simulink model "obs_com_filtro_2020"  (R2020b)
settings: Solver=VariableStepAuto  StartTime=0.0  StopTime=600  RelTol=1e-3
model workspace (MAT data in the model file):
  Td = 2
  std_dev = 0.08
values from neighbouring files (symbols this model uses):
  K = 0.002677    [run_and_calculate.m]
  T = 0.5    [run_and_calculate.m]
libraries: cstblocks x20
settings Model: Creator=Gabriel Vieira  LastModifiedBy=Gabriel Vieira
settings DebuggingCC: SFMachineParentedDataDiag=error

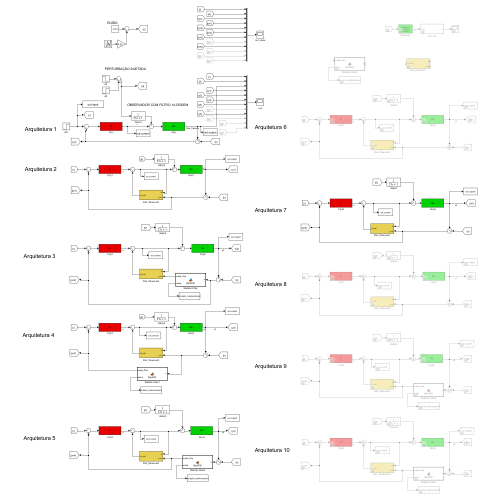
[thumbnail: Simulink's stored preview of the top-level diagram]
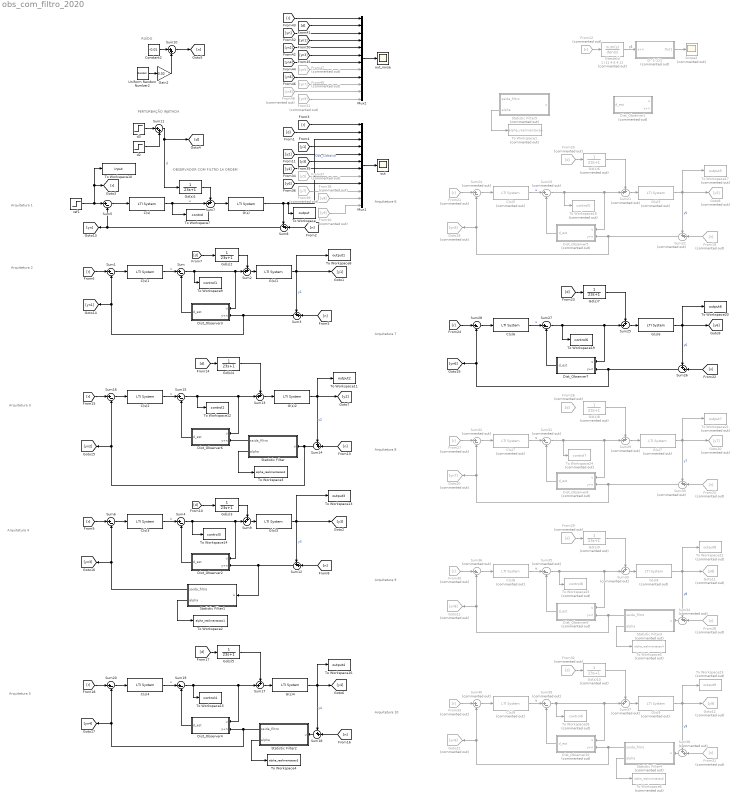
== system obs_com_filtro_2020 ==
  note: RUÍDO
  note: OBSERVADOR COM FILTRO 1A ORDEM
  note: PERTURBAÇÃO INJETADA
  note: Arquitetura 1
  note: Arquitetura 2
  note: Arquitetura 3
  note: Arquitetura 4
  note: Arquitetura 5
  note: Arquitetura 6
  note: Arquitetura 7
  note: Arquitetura 8
  note: Arquitetura 9
  note: Arquitetura 10
  C(s){,1..4,6} (6 alike) : cstblocks/LTI System  sys=C  IC=[]
  C(s){5,7..9} (4 alike) : cstblocks/LTI System  Commented=on  sys=C  IC=[]
  Constant2 : Constant  Value=-0.01
  Dist_Observer1 : Subsystem  Commented=on  mask{std_dev=std_dev}
      mask prompts: std_dev "Noise Std Deviation (std_dev)"
  Dist_Observer10 : Subsystem  Commented=on  mask{Td=Td, std_dev=std_dev}
      mask prompts: Td "Filter time cte (Td)"; std_dev "Noised Std Derivation"
  Dist_Observer2 : Subsystem  mask{Td=Td}
      mask prompts: Td "Filter time cte (Td)"
  Dist_Observer3 : Subsystem  mask{Td=Td}
      mask prompts: Td "Filter time cte (Td)"
  Dist_Observer4 : Subsystem  mask{Td=Td}
      mask prompts: Td "Filter time cte (Td)"
  Dist_Observer5 : Subsystem  Commented=on  mask{Td=Td, std_dev=std_dev}
      mask prompts: Td "Filter time cte (Td)"; std_dev "Noised Std Derivation"
  Dist_Observer6 : Subsystem  mask{Td=Td}
      mask prompts: Td "Filter time cte (Td)"
  Dist_Observer7 : Subsystem  mask{Td=Td, std_dev=std_dev}
      mask prompts: Td "Filter time cte (Td)"; std_dev "Noised Std Derivation"
  Dist_Observer8 : Subsystem  Commented=on  mask{std_dev=std_dev}
      mask prompts: std_dev "Noised Std Derivation"
  Dist_Observer9 : Subsystem  Commented=on  mask{Td=Td, std_dev=std_dev}
      mask prompts: Td "Filter time cte (Td)"; std_dev "Noised Std Derivation"
  From{12,21,27,30,33} (5 alike) : From  Commented=on  GotoTag=r
  From{19,25,28,31} (4 alike) : From  Commented=on  GotoTag=n
  From{20,26,29,32} (4 alike) : From  Commented=on  GotoTag=d
  From37 : From  Commented=on  GotoTag=y5
  From38 : From  Commented=on  GotoTag=y8
  From39 : From  Commented=on  GotoTag=y7
  From40 : From  Commented=on  GotoTag=y9
  From47 : From  Commented=on  GotoTag=yn5
  From48 : From  Commented=on  GotoTag=yn8
  From49 : From  Commented=on  GotoTag=yn7
  From51 : From  Commented=on  GotoTag=yn9
  G(s){,1..4,6} (6 alike) : cstblocks/LTI System  sys=Gs  IC=[]
  G(s){5,7..9} (4 alike) : cstblocks/LTI System  Commented=on  sys=Gs  IC=[]
  "G^{-1}1" : Subsystem  Commented=on
  Gain2 : Gain  Gain=0.02
  Gd(s){1..5,7} (6 alike) : TransferFcn  Numerator=1  Denominator=[23 1]
  Gd(s){6,8..10} (4 alike) : TransferFcn  Commented=on  Numerator=1  Denominator=[23 1]
  Goto10 : Goto  Commented=on  GotoTag=y7
  Goto11 : Goto  Commented=on  GotoTag=y8
  Goto12 : Goto  Commented=on  GotoTag=y9
  Goto18 : Goto  Commented=on  GotoTag=yn5
  Goto20 : Goto  Commented=on  GotoTag=yn7
  Goto21 : Goto  Commented=on  GotoTag=yn8
  Goto22 : Goto  Commented=on  GotoTag=yn9
  Goto8 : Goto  Commented=on  GotoTag=y5
  Gteste(s) : TransferFcn  Commented=on  Numerator=1  Denominator=[1 4 6 4 1]
  Mux1 : Mux  Inputs=12
  Mux2 : Mux  Inputs=12
  Scope2 : Scope  Commented=on
  Statistic Filter : MATLAB Function  TreatAsAtomicUnit=on  mask{std_dev=0.5}
      mask prompts: std_dev "Noise Std Deviation (std_dev)"
  Statistic Filter1 : MATLAB Function  TreatAsAtomicUnit=on  mask{std_dev=0.5}
      mask prompts: std_dev "Noise Std Deviation (std_dev)"
  Statistic Filter2 : MATLAB Function  TreatAsAtomicUnit=on  mask{std_dev=0.5}
      mask prompts: std_dev "Noise Std Deviation (std_dev)"
  Statistic Filter3 : MATLAB Function  Commented=on  TreatAsAtomicUnit=on  mask{std_dev=0.5}
      mask prompts: std_dev "Noise Std Deviation (std_dev)"
  Statistic Filter4 : MATLAB Function  Commented=on  TreatAsAtomicUnit=on  mask{std_dev=0.5}
      mask prompts: std_dev "Noise Std Deviation (std_dev)"
  Statistic Filter5 : MATLAB Function  Commented=on  TreatAsAtomicUnit=on  mask{std_dev=0.5}
      mask prompts: std_dev "Noise Std Deviation (std_dev)"
  Sum{,1,4..6,15..16,19..20,27..28} (11 alike) : Sum  Inputs=|+-
  Sum10 : Sum  Inputs=|++
  Sum11 : Sum  Inputs=|++
  Sum{2..3,7..9,12..14,17..18,25..26} (12 alike) : Sum  Inputs=++|
  Sum{21..22,29..30,33..34,37..38} (8 alike) : Sum  Commented=on  Inputs=++|
  Sum{23..24,31..32,35..36,39..40} (8 alike) : Sum  Commented=on  Inputs=|+-
  To Workspace : ToWorkspace  VariableName=output  SaveFormat=Timeseries  SampleTime=-1
  To Workspace1 : ToWorkspace  Commented=on  VariableName=alpha_realimentacao  SaveFormat=Timeseries  SampleTime=-1
  To Workspace10 : ToWorkspace  VariableName=input  SaveFormat=Timeseries  SampleTime=-1
  To Workspace11 : ToWorkspace  VariableName=output2  SaveFormat=Timeseries  SampleTime=-1
  To Workspace12 : ToWorkspace  VariableName=control2  SaveFormat=Timeseries  SampleTime=-1
  To Workspace13 : ToWorkspace  VariableName=output3  SaveFormat=Timeseries  SampleTime=-1
  To Workspace14 : ToWorkspace  VariableName=control3  SaveFormat=Timeseries  SampleTime=-1
  To Workspace15 : ToWorkspace  VariableName=control4  SaveFormat=Timeseries  SampleTime=-1
  To Workspace16 : ToWorkspace  VariableName=output4  SaveFormat=Timeseries  SampleTime=-1
  To Workspace17 : ToWorkspace  Commented=on  VariableName=output5  SaveFormat=Timeseries  SampleTime=-1
  To Workspace18 : ToWorkspace  Commented=on  VariableName=control5  SaveFormat=Timeseries  SampleTime=-1
  To Workspace19 : ToWorkspace  VariableName=control6  SaveFormat=Timeseries  SampleTime=-1
  To Workspace2 : ToWorkspace  VariableName=alpha_realimentacao1  SaveFormat=Timeseries  SampleTime=-1
  To Workspace20 : ToWorkspace  VariableName=output6  SaveFormat=Timeseries  SampleTime=-1
  To Workspace21 : ToWorkspace  Commented=on  VariableName=output7  SaveFormat=Timeseries  SampleTime=-1
  To Workspace22 : ToWorkspace  Commented=on  VariableName=output8  SaveFormat=Timeseries  SampleTime=-1
  To Workspace23 : ToWorkspace  Commented=on  VariableName=output9  SaveFormat=Timeseries  SampleTime=-1
  To Workspace24 : ToWorkspace  Commented=on  VariableName=control7  SaveFormat=Timeseries  SampleTime=-1
  To Workspace25 : ToWorkspace  Commented=on  VariableName=control8  SaveFormat=Timeseries  SampleTime=-1
  To Workspace26 : ToWorkspace  Commented=on  VariableName=control9  SaveFormat=Timeseries  SampleTime=-1
  To Workspace3 : ToWorkspace  VariableName=alpha_realimentacao2  SaveFormat=Timeseries  SampleTime=-1
  To Workspace4 : ToWorkspace  VariableName=alpha_realimentacao3  SaveFormat=Timeseries  SampleTime=-1
  To Workspace5 : ToWorkspace  Commented=on  VariableName=alpha_realimentacao4  SaveFormat=Timeseries  SampleTime=-1
  To Workspace6 : ToWorkspace  Commented=on  VariableName=alpha_realimentacao6  SaveFormat=Timeseries  SampleTime=-1
  To Workspace7 : ToWorkspace  VariableName=control  SaveFormat=Timeseries  SampleTime=-1
  To Workspace8 : ToWorkspace  VariableName=output1  SaveFormat=Timeseries  SampleTime=-1
  To Workspace9 : ToWorkspace  VariableName=control1  SaveFormat=Timeseries  SampleTime=-1
  Uniform Random Number2 : UniformRandomNumber  SampleTime=0.01
  d2 : Step  Time=150  SampleTime=0
  d3 : Step  Time=200  After=-1  SampleTime=0
  out : Scope
  out_noise : Scope
  ref1 : Step  Time=50  SampleTime=0
  wires:
  Sum10/1 -> [n]
  Constant2/1 -> Sum10/1
  Sum5/1 -> C(s)/1
  d2/1 -> Sum11/2
  C(s)/1 -> To Workspace7/1, Sum7/2  "u"
  Gain2/1 -> Sum10/2
  ref1/1 -> To Workspace10/1, [r], Sum5/1
  Uniform Random Number2/1 -> Gain2/1
  Mux1/1 -> out/1
  Sum7/1 -> G(s)/1
  Sum11/1 -> [d], Gd(s)1/1  "d"
  [r] -> Mux1/1
  Gd(s)1/1 -> Sum7/1
  [n] -> Sum8/2
  d3/1 -> Sum11/1
  G(s)/1 -> Sum8/1, To Workspace/1, Mux1/3  "Obs_Classico"
  Sum8/1 -> [yn], Sum5/2
  [d] -> Mux1/2
  [n] -> Sum3/2
  Gd(s)2/1 -> Sum2/1
  Sum2/1 -> G(s)1/1
  Sum1/1 -> C(s)1/1
  [r] -> Sum1/1
  [d] -> Gd(s)2/1
  C(s)1/1 -> Sum/1  "u"
  Sum/1 -> To Workspace9/1, Dist_Observer3/1(u), Sum2/2
  Sum3/1 -> Dist_Observer3/2(y+n), [yn1], Sum1/2
  Dist_Observer3/1(d_est) -> Sum/2
  G(s)1/1 -> To Workspace8/1, [y1], Sum3/1  "y1"
  [y1] -> Mux1/4
  Statistic Filter5/2(alpha) -> To Workspace1/1
  Sum9/1 -> G(s)3/1
  Gd(s)3/1 -> Sum9/1
  G(s)3/1 -> To Workspace13/1, [y3], Sum12/1  "y3"
  Sum4/1 -> To Workspace14/1, Dist_Observer2/1(u), Sum9/2
  [r] -> Sum6/1
  [d] -> Gd(s)3/1
  C(s)3/1 -> Sum4/1  "u"
  Dist_Observer2/1(d_est) -> Sum4/2
  Sum6/1 -> C(s)3/1
  [n] -> Sum12/2
  Sum12/1 -> Statistic Filter1/1(u), Dist_Observer2/2(y+n)
  Statistic Filter1/2(alpha) -> To Workspace2/1
  [y2] -> Mux1/5
  Gteste(s)/1 -> "G^{-1}1"/1(y+n)  "y1"
  From12/1 -> Gteste(s)/1
  "G^{-1}1"/1(Out1) -> Scope2/1
  Sum15/1 -> To Workspace12/1, Dist_Observer6/1(u), Sum13/2
  [d] -> Gd(s)4/1
  Sum13/1 -> G(s)2/1
  Gd(s)4/1 -> Sum13/1
  [n] -> Sum14/2
  G(s)2/1 -> Sum14/1, To Workspace11/1, [y2]  "y2"
  Statistic Filter/2(alpha) -> To Workspace3/1
  Sum16/1 -> C(s)2/1
  Dist_Observer6/1(d_est) -> Sum15/2
  C(s)2/1 -> Sum15/1  "u"
  Statistic Filter/1(saida_filtro) -> Dist_Observer6/2(y+n)
  [r] -> Sum16/1
  Dist_Observer4/1(d_est) -> Sum19/2
  [r] -> Sum20/1
  Sum17/1 -> G(s)4/1
  Sum18/1 -> Statistic Filter2/1(u)
  Statistic Filter2/2(alpha) -> To Workspace4/1
  G(s)4/1 -> To Workspace16/1, [y4], Sum18/1  "y4"
  [d] -> Gd(s)5/1
  Sum20/1 -> C(s)4/1
  C(s)4/1 -> Sum19/1  "u"
  Sum19/1 -> To Workspace15/1, Dist_Observer4/1(u), Sum17/2
  Gd(s)5/1 -> Sum17/1
  [n] -> Sum18/2
  Sum23/1 -> To Workspace18/1, Dist_Observer5/1(u), Sum21/2
  From19/1 -> Sum22/2
  Gd(s)6/1 -> Sum21/1
  Sum24/1 -> C(s)5/1
  From20/1 -> Gd(s)6/1
  C(s)5/1 -> Sum23/1  "u"
  G(s)5/1 -> To Workspace17/1, Goto8/1, Sum22/1  "y5"
  Dist_Observer5/1(d_est) -> Sum23/2
  Sum21/1 -> G(s)5/1
  From21/1 -> Sum24/1
  Gd(s)7/1 -> Sum25/1
  Sum27/1 -> To Workspace19/1, Dist_Observer7/1(u), Sum25/2
  [n] -> Sum26/2
  G(s)6/1 -> To Workspace20/1, [y6], Sum26/1  "y6"
  Sum28/1 -> C(s)6/1
  C(s)6/1 -> Sum27/1  "u"
  [r] -> Sum28/1
  Dist_Observer7/1(d_est) -> Sum27/2
  [d] -> Gd(s)7/1
  Sum25/1 -> G(s)6/1
  Sum31/1 -> Dist_Observer8/1(u), Sum29/2, To Workspace24/1
  Gd(s)8/1 -> Sum29/1
  Dist_Observer8/1(d_est) -> Sum31/2
  From27/1 -> Sum32/1
  C(s)7/1 -> Sum31/1  "u"
  Sum32/1 -> C(s)7/1
  From25/1 -> Sum30/2
  G(s)7/1 -> To Workspace21/1, Goto10/1, Sum30/1  "y7"
  Sum29/1 -> G(s)7/1
  Sum38/1 -> Statistic Filter4/1(u)
  Statistic Filter4/2(alpha) -> To Workspace6/1
  Sum39/1 -> To Workspace26/1, Dist_Observer10/1(u), Sum37/2
  Gd(s)10/1 -> Sum37/1
  Dist_Observer10/1(d_est) -> Sum39/2
  G(s)9/1 -> To Workspace23/1, Goto12/1, Sum38/1  "y9"
  From31/1 -> Sum38/2
  Sum34/1 -> Statistic Filter3/1(u)
  Sum40/1 -> C(s)9/1
  C(s)9/1 -> Sum39/1  "u"
  Statistic Filter3/2(alpha) -> To Workspace5/1
  Gd(s)9/1 -> Sum33/1
  Sum35/1 -> To Workspace25/1, Dist_Observer9/1(u), Sum33/2
  From28/1 -> Sum34/2
  G(s)8/1 -> To Workspace22/1, Goto11/1, Sum34/1  "y8"
  From30/1 -> Sum36/1
  From33/1 -> Sum40/1
  Dist_Observer9/1(d_est) -> Sum35/2
  From29/1 -> Gd(s)9/1
  Sum33/1 -> G(s)8/1
  Sum37/1 -> G(s)9/1
  Sum36/1 -> C(s)8/1
  C(s)8/1 -> Sum35/1  "u"
  From32/1 -> Gd(s)10/1
  [y3] -> Mux1/6
  [y4] -> Mux1/7
  From37/1 -> Mux1/8
  [y6] -> Mux1/9
  From39/1 -> Mux1/10
  From38/1 -> Mux1/11
  From40/1 -> Mux1/12
  From51/1 -> Mux2/12
  From48/1 -> Mux2/11
  [yn6] -> Mux2/9
  From49/1 -> Mux2/10
  [yn3] -> Mux2/6
  [yn1] -> Mux2/4
  From47/1 -> Mux2/8
  [r] -> Mux2/1
  [yn4] -> Mux2/7
  [d] -> Mux2/2
  Mux2/1 -> out_noise/1
  [yn2] -> Mux2/5
  [yn] -> Mux2/3
  Sum14/1 -> Statistic Filter/1(u), [yn2], Sum16/2
  Statistic Filter1/1(saida_filtro) -> [yn3], Sum6/2
  Statistic Filter2/1(saida_filtro) -> Dist_Observer4/2(y+n), [yn4], Sum20/2
  Sum22/1 -> Dist_Observer5/2(y+n), Goto18/1, Sum24/2
  Sum26/1 -> Dist_Observer7/2(y+n), [yn6], Sum28/2
  Sum30/1 -> Dist_Observer8/2(y+n), Goto20/1, Sum32/2
  Statistic Filter3/1(saida_filtro) -> Dist_Observer9/2(y+n), Goto21/1, Sum36/2
  Statistic Filter4/1(saida_filtro) -> Dist_Observer10/2(y+n), Goto22/1, Sum40/2

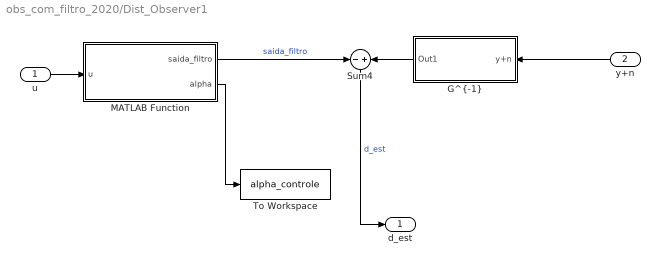
== system obs_com_filtro_2020/Dist_Observer1 ==
  u : Inport
  y+n : Inport  Port=2
  "G^{-1}" : Subsystem
  MATLAB Function : MATLAB Function  TreatAsAtomicUnit=on
  Sum4 : Sum  Inputs=-|+
  To Workspace : ToWorkspace  VariableName=alpha_controle  SaveFormat=Timeseries  SampleTime=-1
  d_est : Outport
  wires:
  MATLAB Function/1(saida_filtro) -> Sum4/1  "saida_filtro"
  Sum4/1 -> d_est/1  "d_est"
  u/1 -> MATLAB Function/1(u)
  "G^{-1}"/1(Out1) -> Sum4/2
  MATLAB Function/2(alpha) -> To Workspace/1
  y+n/1 -> "G^{-1}"/1(y+n)

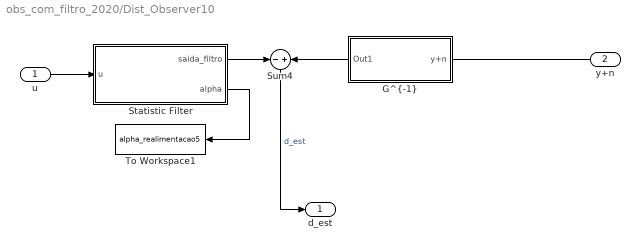
== system obs_com_filtro_2020/Dist_Observer10 ==
  u : Inport
  y+n : Inport  Port=2
  "G^{-1}" : Subsystem
  Statistic Filter : MATLAB Function  TreatAsAtomicUnit=on  mask{std_dev=0.5}
      mask prompts: std_dev "Noise Std Deviation (std_dev)"
  Sum4 : Sum  Inputs=-|+
  To Workspace1 : ToWorkspace  VariableName=alpha_realimentacao5  SaveFormat=Timeseries  SampleTime=-1
  d_est : Outport
  wires:
  Statistic Filter/1(saida_filtro) -> Sum4/1
  Sum4/1 -> d_est/1  "d_est"
  u/1 -> Statistic Filter/1(u)
  "G^{-1}"/1(Out1) -> Sum4/2
  y+n/1 -> ?
  Statistic Filter/2(alpha) -> To Workspace1/1

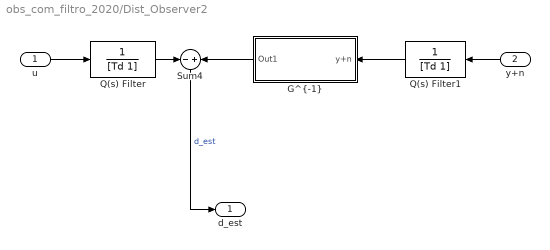
== system obs_com_filtro_2020/Dist_Observer2 ==
  u : Inport
  y+n : Inport  Port=2
  "G^{-1}" : Subsystem
  Q(s) Filter : TransferFcn  Denominator=[Td 1]
  Q(s) Filter1 : TransferFcn  Denominator=[Td 1]
  Sum4 : Sum  Inputs=-|+
  d_est : Outport
  wires:
  Q(s) Filter/1 -> Sum4/1
  Sum4/1 -> d_est/1  "d_est"
  u/1 -> Q(s) Filter/1
  "G^{-1}"/1(Out1) -> Sum4/2
  Q(s) Filter1/1 -> "G^{-1}"/1(y+n)
  y+n/1 -> Q(s) Filter1/1

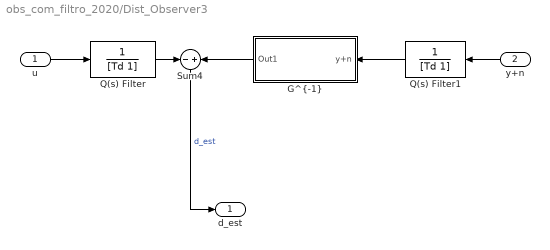
== system obs_com_filtro_2020/Dist_Observer3 ==
  u : Inport
  y+n : Inport  Port=2
  "G^{-1}" : Subsystem
  Q(s) Filter : TransferFcn  Denominator=[Td 1]
  Q(s) Filter1 : TransferFcn  Denominator=[Td 1]
  Sum4 : Sum  Inputs=-|+
  d_est : Outport
  wires:
  Q(s) Filter/1 -> Sum4/1
  Sum4/1 -> d_est/1  "d_est"
  u/1 -> Q(s) Filter/1
  "G^{-1}"/1(Out1) -> Sum4/2
  Q(s) Filter1/1 -> "G^{-1}"/1(y+n)
  y+n/1 -> Q(s) Filter1/1

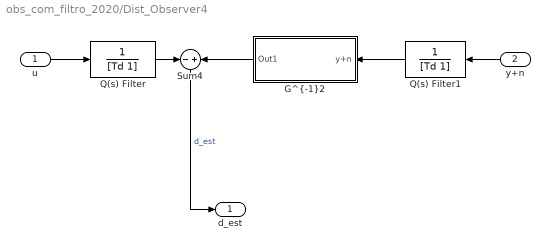
== system obs_com_filtro_2020/Dist_Observer4 ==
  u : Inport
  y+n : Inport  Port=2
  "G^{-1}2" : Subsystem
  Q(s) Filter : TransferFcn  Denominator=[Td 1]
  Q(s) Filter1 : TransferFcn  Denominator=[Td 1]
  Sum4 : Sum  Inputs=-|+
  d_est : Outport
  wires:
  Q(s) Filter/1 -> Sum4/1
  Sum4/1 -> d_est/1  "d_est"
  u/1 -> Q(s) Filter/1
  "G^{-1}2"/1(Out1) -> Sum4/2
  Q(s) Filter1/1 -> "G^{-1}2"/1(y+n)
  y+n/1 -> Q(s) Filter1/1

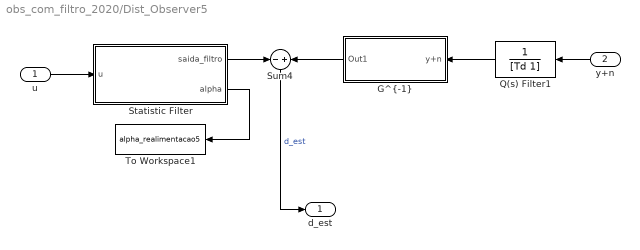
== system obs_com_filtro_2020/Dist_Observer5 ==
  u : Inport
  y+n : Inport  Port=2
  "G^{-1}" : Subsystem
  Q(s) Filter1 : TransferFcn  Denominator=[Td 1]
  Statistic Filter : MATLAB Function  TreatAsAtomicUnit=on  mask{std_dev=0.5}
      mask prompts: std_dev "Noise Std Deviation (std_dev)"
  Sum4 : Sum  Inputs=-|+
  To Workspace1 : ToWorkspace  VariableName=alpha_realimentacao5  SaveFormat=Timeseries  SampleTime=-1
  d_est : Outport
  wires:
  Statistic Filter/1(saida_filtro) -> Sum4/1
  Sum4/1 -> d_est/1  "d_est"
  u/1 -> Statistic Filter/1(u)
  "G^{-1}"/1(Out1) -> Sum4/2
  Q(s) Filter1/1 -> "G^{-1}"/1(y+n)
  y+n/1 -> Q(s) Filter1/1
  Statistic Filter/2(alpha) -> To Workspace1/1

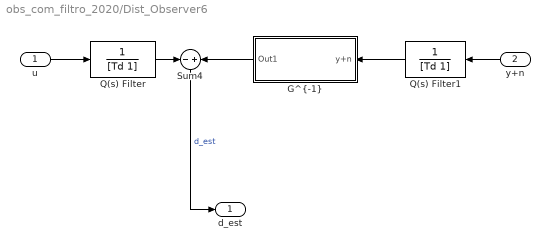
== system obs_com_filtro_2020/Dist_Observer6 ==
  u : Inport
  y+n : Inport  Port=2
  "G^{-1}" : Subsystem
  Q(s) Filter : TransferFcn  Denominator=[Td 1]
  Q(s) Filter1 : TransferFcn  Denominator=[Td 1]
  Sum4 : Sum  Inputs=-|+
  d_est : Outport
  wires:
  Q(s) Filter/1 -> Sum4/1
  Sum4/1 -> d_est/1  "d_est"
  u/1 -> Q(s) Filter/1
  "G^{-1}"/1(Out1) -> Sum4/2
  Q(s) Filter1/1 -> "G^{-1}"/1(y+n)
  y+n/1 -> Q(s) Filter1/1

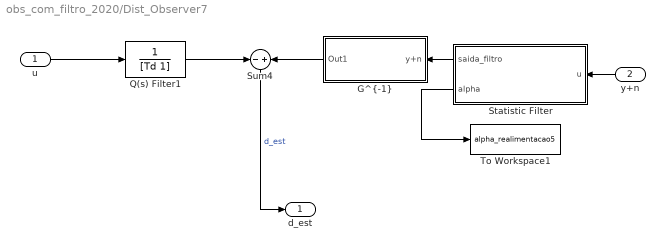
== system obs_com_filtro_2020/Dist_Observer7 ==
  u : Inport
  y+n : Inport  Port=2
  "G^{-1}" : Subsystem
  Q(s) Filter1 : TransferFcn  Denominator=[Td 1]
  Statistic Filter : MATLAB Function  TreatAsAtomicUnit=on  mask{std_dev=0.5}
      mask prompts: std_dev "Noise Std Deviation (std_dev)"
  Sum4 : Sum  Inputs=-|+
  To Workspace1 : ToWorkspace  VariableName=alpha_realimentacao5  SaveFormat=Timeseries  SampleTime=-1
  d_est : Outport
  wires:
  Sum4/1 -> d_est/1  "d_est"
  "G^{-1}"/1(Out1) -> Sum4/2
  Statistic Filter/2(alpha) -> To Workspace1/1
  Q(s) Filter1/1 -> Sum4/1
  u/1 -> Q(s) Filter1/1
  Statistic Filter/1(saida_filtro) -> "G^{-1}"/1(y+n)
  y+n/1 -> Statistic Filter/1(u)

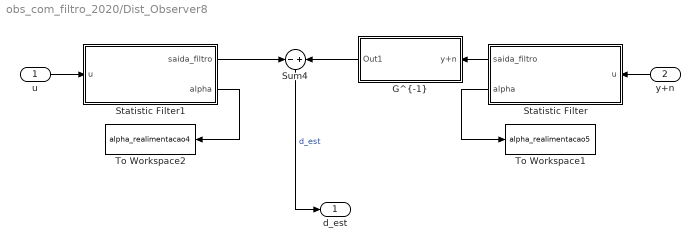
== system obs_com_filtro_2020/Dist_Observer8 ==
  u : Inport
  y+n : Inport  Port=2
  "G^{-1}" : Subsystem
  Statistic Filter : MATLAB Function  TreatAsAtomicUnit=on  mask{std_dev=0.5}
      mask prompts: std_dev "Noise Std Deviation (std_dev)"
  Statistic Filter1 : MATLAB Function  TreatAsAtomicUnit=on  mask{std_dev=0.5}
      mask prompts: std_dev "Noise Std Deviation (std_dev)"
  Sum4 : Sum  Inputs=-|+
  To Workspace1 : ToWorkspace  VariableName=alpha_realimentacao5  SaveFormat=Timeseries  SampleTime=-1
  To Workspace2 : ToWorkspace  VariableName=alpha_realimentacao4  SaveFormat=Timeseries  SampleTime=-1
  d_est : Outport
  wires:
  Sum4/1 -> d_est/1  "d_est"
  "G^{-1}"/1(Out1) -> Sum4/2
  Statistic Filter/2(alpha) -> To Workspace1/1
  Statistic Filter1/1(saida_filtro) -> Sum4/1
  u/1 -> Statistic Filter1/1(u)
  Statistic Filter/1(saida_filtro) -> "G^{-1}"/1(y+n)
  y+n/1 -> Statistic Filter/1(u)
  Statistic Filter1/2(alpha) -> To Workspace2/1

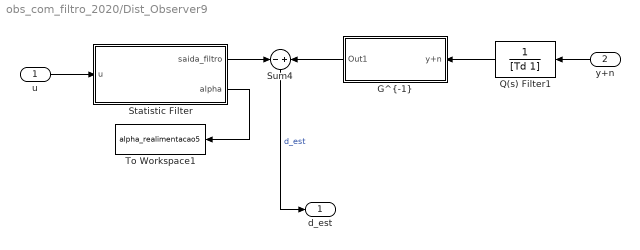
== system obs_com_filtro_2020/Dist_Observer9 ==
  u : Inport
  y+n : Inport  Port=2
  "G^{-1}" : Subsystem
  Q(s) Filter1 : TransferFcn  Denominator=[Td 1]
  Statistic Filter : MATLAB Function  TreatAsAtomicUnit=on  mask{std_dev=0.5}
      mask prompts: std_dev "Noise Std Deviation (std_dev)"
  Sum4 : Sum  Inputs=-|+
  To Workspace1 : ToWorkspace  VariableName=alpha_realimentacao5  SaveFormat=Timeseries  SampleTime=-1
  d_est : Outport
  wires:
  Statistic Filter/1(saida_filtro) -> Sum4/1
  Sum4/1 -> d_est/1  "d_est"
  u/1 -> Statistic Filter/1(u)
  "G^{-1}"/1(Out1) -> Sum4/2
  Q(s) Filter1/1 -> "G^{-1}"/1(y+n)
  y+n/1 -> Q(s) Filter1/1
  Statistic Filter/2(alpha) -> To Workspace1/1

== system obs_com_filtro_2020/G^{-1}1 ==
  y+n : Inport
  Derivative : Derivative  CoefficientInTFapproximation=1e-6
  Sum : Sum  Inputs=|++
  Out1 : Outport
  wires:
  Derivative/1 -> Sum/2
  Sum/1 -> Out1/1
  y+n/1 -> Derivative/1, Sum/1

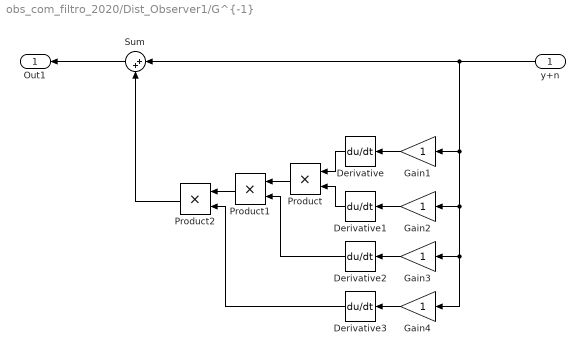
== system obs_com_filtro_2020/Dist_Observer1/G^{-1} ==
  y+n : Inport
  Derivative{,1..3} (4 alike) : Derivative  CoefficientInTFapproximation=1e-6
  Gain{1..4} (4 alike) : Gain
  Product : Product
  Product1 : Product
  Product2 : Product
  Sum : Sum  Inputs=|++
  Out1 : Outport
  wires:
  Sum/1 -> Out1/1
  Gain1/1 -> Derivative/1
  Derivative/1 -> Product/1
  Gain2/1 -> Derivative1/1
  Derivative1/1 -> Product/2
  Gain3/1 -> Derivative2/1
  y+n/1 -> Sum/1, Gain4/1, Gain3/1, Gain2/1, Gain1/1
  Gain4/1 -> Derivative3/1
  Product/1 -> Product1/1
  Derivative2/1 -> Product1/2
  Product1/1 -> Product2/1
  Derivative3/1 -> Product2/2
  Product2/1 -> Sum/2

== system obs_com_filtro_2020/Dist_Observer10/G^{-1} ==
  y+n : Inport
  Derivative : Derivative  CoefficientInTFapproximation=1e-6
  Gain : Gain  Gain=1/K
  Gain1 : Gain  Gain=T
  Sum : Sum  Inputs=|++
  Out1 : Outport
  wires:
  Gain/1 -> Gain1/1, Sum/1
  Sum/1 -> Out1/1
  Derivative/1 -> Sum/2
  Gain1/1 -> Derivative/1
  y+n/1 -> Gain/1

== system obs_com_filtro_2020/Dist_Observer2/G^{-1} ==
  y+n : Inport
  Derivative : Derivative  CoefficientInTFapproximation=1e-6
  Gain : Gain  Gain=1/K
  Gain1 : Gain  Gain=T
  Sum : Sum  Inputs=|++
  Out1 : Outport
  wires:
  Gain/1 -> Gain1/1, Sum/1
  Sum/1 -> Out1/1
  Derivative/1 -> Sum/2
  Gain1/1 -> Derivative/1
  y+n/1 -> Gain/1

== system obs_com_filtro_2020/Dist_Observer3/G^{-1} ==
  y+n : Inport
  Derivative : Derivative  CoefficientInTFapproximation=1e-6
  Gain : Gain  Gain=1/K
  Gain1 : Gain  Gain=T
  Sum : Sum  Inputs=|++
  Out1 : Outport
  wires:
  Gain/1 -> Gain1/1, Sum/1
  Sum/1 -> Out1/1
  Derivative/1 -> Sum/2
  Gain1/1 -> Derivative/1
  y+n/1 -> Gain/1

== system obs_com_filtro_2020/Dist_Observer4/G^{-1}2 ==
  y+n : Inport
  Derivative : Derivative  CoefficientInTFapproximation=1e-6
  Sum : Sum  Inputs=|++
  Out1 : Outport
  wires:
  Derivative/1 -> Sum/2
  Sum/1 -> Out1/1
  y+n/1 -> Derivative/1, Sum/1

== system obs_com_filtro_2020/Dist_Observer5/G^{-1} ==
  y+n : Inport
  Derivative : Derivative  CoefficientInTFapproximation=1e-6
  Gain : Gain  Gain=1/K
  Gain1 : Gain  Gain=T
  Sum : Sum  Inputs=|++
  Out1 : Outport
  wires:
  Gain/1 -> Gain1/1, Sum/1
  Sum/1 -> Out1/1
  Derivative/1 -> Sum/2
  Gain1/1 -> Derivative/1
  y+n/1 -> Gain/1

== system obs_com_filtro_2020/Dist_Observer6/G^{-1} ==
  y+n : Inport
  Derivative : Derivative  CoefficientInTFapproximation=1e-6
  Gain : Gain  Gain=1/K
  Gain1 : Gain  Gain=T
  Sum : Sum  Inputs=|++
  Out1 : Outport
  wires:
  Gain/1 -> Gain1/1, Sum/1
  Sum/1 -> Out1/1
  Derivative/1 -> Sum/2
  Gain1/1 -> Derivative/1
  y+n/1 -> Gain/1

== system obs_com_filtro_2020/Dist_Observer7/G^{-1} ==
  y+n : Inport
  Derivative : Derivative  CoefficientInTFapproximation=1e-6
  Gain : Gain  Gain=1/K
  Gain1 : Gain  Gain=T
  Sum : Sum  Inputs=|++
  Out1 : Outport
  wires:
  Gain/1 -> Gain1/1, Sum/1
  Sum/1 -> Out1/1
  Derivative/1 -> Sum/2
  Gain1/1 -> Derivative/1
  y+n/1 -> Gain/1

== system obs_com_filtro_2020/Dist_Observer8/G^{-1} ==
  y+n : Inport
  Derivative : Derivative  CoefficientInTFapproximation=1e-6
  Gain : Gain  Gain=1/K
  Gain1 : Gain  Gain=T
  Sum : Sum  Inputs=|++
  Out1 : Outport
  wires:
  Gain/1 -> Gain1/1, Sum/1
  Sum/1 -> Out1/1
  Derivative/1 -> Sum/2
  Gain1/1 -> Derivative/1
  y+n/1 -> Gain/1

== system obs_com_filtro_2020/Dist_Observer9/G^{-1} ==
  y+n : Inport
  Derivative : Derivative  CoefficientInTFapproximation=1e-6
  Gain : Gain  Gain=1/K
  Gain1 : Gain  Gain=T
  Sum : Sum  Inputs=|++
  Out1 : Outport
  wires:
  Gain/1 -> Gain1/1, Sum/1
  Sum/1 -> Out1/1
  Derivative/1 -> Sum/2
  Gain1/1 -> Derivative/1
  y+n/1 -> Gain/1

== matlab function obs_com_filtro_2020/Dist_Observer9/Statistic Filter ==
  settings: updateMethod=DISCRETE
  data: u input; saida_filtro output; std_dev parameter; alpha output
%Autor: Lucas Moura Gomes
%Filtro estatístico.

function [saida_filtro, alpha]  = filtroPID( u, std_dev)
    persistent x_ant;
    persistent alpha_orig;
    
    if isempty(x_ant)
        x_ant = 0;
        Ts = 0.01; %sampling time
        tf = 2; %continuous time cte.
        alpha_orig = 1 - exp(-1/tf * Ts); %c2d filter
    end
    
    alpha = erf(abs(x_ant - u)/(sqrt(2)*2*std_dev));
    
    if alpha > 1
        alpha = 1;
    end
    
    %up = 1.1; %upper bound 10%
    %alpha = alpha * alpha_orig * up;
    
    saida_filtro = (1-alpha)*x_ant + alpha*u;
    
    x_ant = saida_filtro;
end

%Autor: Lucas Moura Gomes
%Filtro estatístico.
% 
% function [saida_filtro, alpha] = filtroPID( u, erro_tipico_medicao, Tf  )
% 	
%     persistent x_ant;
%     
%     if isempty(x_ant)
%         x_ant = 0;
%     end
%     
%     Tf = Tf/1.5;
%     a_Tf = 1 - exp(-1/Tf * 5);
%     
%     alpha = erf(abs(x_ant - u)/(sqrt(2)*2*erro_tipico_medicao));
%     
%     if alpha > 1 
%         alpha = 1;
%     end;
%     
%     saida_filtro = (1-alpha)*x_ant + alpha*u;
% 
%     x_ant = saida_filtro;
%         
% 
%     saida_filtro = x_ant;
% 
%     
% end

== matlab function obs_com_filtro_2020/Statistic Filter4 ==
  settings: updateMethod=DISCRETE
  data: u input; saida_filtro output; std_dev parameter; alpha output
%Autor: Lucas Moura Gomes
%Filtro estatístico.

function [saida_filtro, alpha]  = filtroPID( u, std_dev)
    persistent x_ant;
    persistent alpha_orig;
    
    if isempty(x_ant)
        x_ant = 0;
        Ts = 0.01; %sampling time
        tf = 2; %continuous time cte.
        alpha_orig = 1 - exp(-1/tf * Ts); %c2d filter
    end
    
    alpha = erf(abs(x_ant - u)/(sqrt(2)*2*std_dev));
    
    if alpha > 1
        alpha = 1;
    end
    
    %up = 1.1; %upper bound 10%
    %alpha = alpha * alpha_orig * up;
    
    saida_filtro = (1-alpha)*x_ant + alpha*u;
    
    x_ant = saida_filtro;
end

%Autor: Lucas Moura Gomes
%Filtro estatístico.
% 
% function [saida_filtro, alpha] = filtroPID( u, erro_tipico_medicao, Tf  )
% 	
%     persistent x_ant;
%     
%     if isempty(x_ant)
%         x_ant = 0;
%     end
%     
%     Tf = Tf/1.5;
%     a_Tf = 1 - exp(-1/Tf * 5);
%     
%     alpha = erf(abs(x_ant - u)/(sqrt(2)*2*erro_tipico_medicao));
%     
%     if alpha > 1 
%         alpha = 1;
%     end;
%     
%     saida_filtro = (1-alpha)*x_ant + alpha*u;
% 
%     x_ant = saida_filtro;
%         
% 
%     saida_filtro = x_ant;
% 
%     
% end

== matlab function obs_com_filtro_2020/Statistic Filter1 ==
  settings: updateMethod=DISCRETE
  data: u input; saida_filtro output; std_dev parameter; alpha output
%Autor: Lucas Moura Gomes
%Filtro estatístico.

function [saida_filtro, alpha]  = filtroPID( u, std_dev)
    persistent x_ant;
    persistent alpha_orig;
    
    if isempty(x_ant)
        x_ant = 0;
        Ts = 0.01; %sampling time
        tf = 2; %continuous time cte.
        alpha_orig = 1 - exp(-1/tf * Ts); %c2d filter
    end
    
    alpha = erf(abs(x_ant - u)/(sqrt(2)*2*std_dev));
    
    if alpha > 1
        alpha = 1;
    end
    
    %up = 1.1; %upper bound 10%
    %alpha = alpha * alpha_orig * up;
    
    saida_filtro = (1-alpha)*x_ant + alpha*u;
    
    x_ant = saida_filtro;
end

%Autor: Lucas Moura Gomes
%Filtro estatístico.
% 
% function [saida_filtro, alpha] = filtroPID( u, erro_tipico_medicao, Tf  )
% 	
%     persistent x_ant;
%     
%     if isempty(x_ant)
%         x_ant = 0;
%     end
%     
%     Tf = Tf/1.5;
%     a_Tf = 1 - exp(-1/Tf * 5);
%     
%     alpha = erf(abs(x_ant - u)/(sqrt(2)*2*erro_tipico_medicao));
%     
%     if alpha > 1 
%         alpha = 1;
%     end;
%     
%     saida_filtro = (1-alpha)*x_ant + alpha*u;
% 
%     x_ant = saida_filtro;
%         
% 
%     saida_filtro = x_ant;
% 
%     
% end

== matlab function obs_com_filtro_2020/Statistic Filter2 ==
  settings: updateMethod=DISCRETE
  data: u input; saida_filtro output; std_dev parameter; alpha output
%Autor: Lucas Moura Gomes
%Filtro estatístico.

function [saida_filtro, alpha]  = filtroPID( u, std_dev)
    persistent x_ant;
    persistent alpha_orig;
    
    if isempty(x_ant)
        x_ant = 0;
        Ts = 0.01; %sampling time
        tf = 2; %continuous time cte.
        alpha_orig = 1 - exp(-1/tf * Ts); %c2d filter
    end
    
    alpha = erf(abs(x_ant - u)/(sqrt(2)*2*std_dev));
    
    if alpha > 1
        alpha = 1;
    end
    
    %up = 1.1; %upper bound 10%
    %alpha = alpha * alpha_orig * up;
    
    saida_filtro = (1-alpha)*x_ant + alpha*u;
    
    x_ant = saida_filtro;
end

%Autor: Lucas Moura Gomes
%Filtro estatístico.
% 
% function [saida_filtro, alpha] = filtroPID( u, erro_tipico_medicao, Tf  )
% 	
%     persistent x_ant;
%     
%     if isempty(x_ant)
%         x_ant = 0;
%     end
%     
%     Tf = Tf/1.5;
%     a_Tf = 1 - exp(-1/Tf * 5);
%     
%     alpha = erf(abs(x_ant - u)/(sqrt(2)*2*erro_tipico_medicao));
%     
%     if alpha > 1 
%         alpha = 1;
%     end;
%     
%     saida_filtro = (1-alpha)*x_ant + alpha*u;
% 
%     x_ant = saida_filtro;
%         
% 
%     saida_filtro = x_ant;
% 
%     
% end

== matlab function obs_com_filtro_2020/Dist_Observer1/MATLAB Function ==
  settings: updateMethod=DISCRETE
  data: u input; saida_filtro output; std_dev parameter; alpha output
%Autor: Lucas Moura Gomes
%Filtro estatístico.

function [saida_filtro, alpha]  = filtroPID( u, std_dev)
    persistent x_ant;
    persistent alpha_orig;
    
    if isempty(x_ant)
        x_ant = 0;
        alpha_orig = 1 - exp(-1/2 * 0.01);
    end;
    
    alpha = erf(abs(x_ant - u)/(sqrt(2)*2*std_dev));
    
    if alpha > 1
        alpha = 1;
    end;
    
    alpha = alpha * alpha_orig * 1.1;
    
    saida_filtro = (1-alpha)*x_ant + alpha*u;
    
    x_ant = saida_filtro;
end

== matlab function obs_com_filtro_2020/Statistic Filter5 ==
  settings: updateMethod=DISCRETE
  data: u input; saida_filtro output; std_dev parameter; alpha output
%Autor: Lucas Moura Gomes
%Filtro estatístico.

function [saida_filtro, alpha]  = filtroPID( u, std_dev)
    persistent x_ant;
    persistent alpha_orig;
    
    if isempty(x_ant)
        x_ant = 0;
        Ts = 0.01; %sampling time
        tf = 2; %continuous time cte.
        alpha_orig = 1 - exp(-1/tf * Ts); %c2d filter
    end
    
    alpha = erf(abs(x_ant - u)/(sqrt(2)*2*std_dev));
    
    if alpha > 1
        alpha = 1;
    end
    
    %up = 1.1; %upper bound 10%
    %alpha = alpha * alpha_orig * up;
    
    saida_filtro = (1-alpha)*x_ant + alpha*u;
    
    x_ant = saida_filtro;
end

%Autor: Lucas Moura Gomes
%Filtro estatístico.
% 
% function [saida_filtro, alpha] = filtroPID( u, erro_tipico_medicao, Tf  )
% 	
%     persistent x_ant;
%     
%     if isempty(x_ant)
%         x_ant = 0;
%     end
%     
%     Tf = Tf/1.5;
%     a_Tf = 1 - exp(-1/Tf * 5);
%     
%     alpha = erf(abs(x_ant - u)/(sqrt(2)*2*erro_tipico_medicao));
%     
%     if alpha > 1 
%         alpha = 1;
%     end;
%     
%     saida_filtro = (1-alpha)*x_ant + alpha*u;
% 
%     x_ant = saida_filtro;
%         
% 
%     saida_filtro = x_ant;
% 
%     
% end

== matlab function obs_com_filtro_2020/Statistic Filter ==
  settings: updateMethod=DISCRETE
  data: u input; saida_filtro output; std_dev parameter; alpha output
%Autor: Lucas Moura Gomes
%Filtro estatístico.

function [saida_filtro, alpha]  = filtroPID( u, std_dev)
    persistent x_ant;
    persistent alpha_orig;
    
    if isempty(x_ant)
        x_ant = 0;
        Ts = 0.01; %sampling time
        tf = 2; %continuous time cte.
        alpha_orig = 1 - exp(-1/tf * Ts); %c2d filter
    end
    
    alpha = erf(abs(x_ant - u)/(sqrt(2)*2*std_dev));
    
    if alpha > 1
        alpha = 1;
    end
    
    %up = 1.1; %upper bound 10%
    %alpha = alpha * alpha_orig * up;
    
    saida_filtro = (1-alpha)*x_ant + alpha*u;
    
    x_ant = saida_filtro;
end

%Autor: Lucas Moura Gomes
%Filtro estatístico.
% 
% function [saida_filtro, alpha] = filtroPID( u, erro_tipico_medicao, Tf  )
% 	
%     persistent x_ant;
%     
%     if isempty(x_ant)
%         x_ant = 0;
%     end
%     
%     Tf = Tf/1.5;
%     a_Tf = 1 - exp(-1/Tf * 5);
%     
%     alpha = erf(abs(x_ant - u)/(sqrt(2)*2*erro_tipico_medicao));
%     
%     if alpha > 1 
%         alpha = 1;
%     end;
%     
%     saida_filtro = (1-alpha)*x_ant + alpha*u;
% 
%     x_ant = saida_filtro;
%         
% 
%     saida_filtro = x_ant;
% 
%     
% end

== matlab function obs_com_filtro_2020/Statistic Filter3 ==
  settings: updateMethod=DISCRETE
  data: u input; saida_filtro output; std_dev parameter; alpha output
%Autor: Lucas Moura Gomes
%Filtro estatístico.

function [saida_filtro, alpha]  = filtroPID( u, std_dev)
    persistent x_ant;
    persistent alpha_orig;
    
    if isempty(x_ant)
        x_ant = 0;
        Ts = 0.01; %sampling time
        tf = 2; %continuous time cte.
        alpha_orig = 1 - exp(-1/tf * Ts); %c2d filter
    end
    
    alpha = erf(abs(x_ant - u)/(sqrt(2)*2*std_dev));
    
    if alpha > 1
        alpha = 1;
    end
    
    %up = 1.1; %upper bound 10%
    %alpha = alpha * alpha_orig * up;
    
    saida_filtro = (1-alpha)*x_ant + alpha*u;
    
    x_ant = saida_filtro;
end

%Autor: Lucas Moura Gomes
%Filtro estatístico.
% 
% function [saida_filtro, alpha] = filtroPID( u, erro_tipico_medicao, Tf  )
% 	
%     persistent x_ant;
%     
%     if isempty(x_ant)
%         x_ant = 0;
%     end
%     
%     Tf = Tf/1.5;
%     a_Tf = 1 - exp(-1/Tf * 5);
%     
%     alpha = erf(abs(x_ant - u)/(sqrt(2)*2*erro_tipico_medicao));
%     
%     if alpha > 1 
%         alpha = 1;
%     end;
%     
%     saida_filtro = (1-alpha)*x_ant + alpha*u;
% 
%     x_ant = saida_filtro;
%         
% 
%     saida_filtro = x_ant;
% 
%     
% end

== matlab function obs_com_filtro_2020/Dist_Observer8/Statistic Filter ==
  settings: updateMethod=DISCRETE
  data: u input; saida_filtro output; std_dev parameter; alpha output
%Autor: Lucas Moura Gomes
%Filtro estatístico.

function [saida_filtro, alpha]  = filtroPID( u, std_dev)
    persistent x_ant;
    persistent alpha_orig;
    
    if isempty(x_ant)
        x_ant = 0;
        Ts = 0.01; %sampling time
        tf = 2; %continuous time cte.
        alpha_orig = 1 - exp(-1/tf * Ts); %c2d filter
    end
    
    alpha = erf(abs(x_ant - u)/(sqrt(2)*2*std_dev));
    
    if alpha > 1
        alpha = 1;
    end
    
    %up = 1.1; %upper bound 10%
    %alpha = alpha * alpha_orig * up;
    
    saida_filtro = (1-alpha)*x_ant + alpha*u;
    
    x_ant = saida_filtro;
end

%Autor: Lucas Moura Gomes
%Filtro estatístico.
% 
% function [saida_filtro, alpha] = filtroPID( u, erro_tipico_medicao, Tf  )
% 	
%     persistent x_ant;
%     
%     if isempty(x_ant)
%         x_ant = 0;
%     end
%     
%     Tf = Tf/1.5;
%     a_Tf = 1 - exp(-1/Tf * 5);
%     
%     alpha = erf(abs(x_ant - u)/(sqrt(2)*2*erro_tipico_medicao));
%     
%     if alpha > 1 
%         alpha = 1;
%     end;
%     
%     saida_filtro = (1-alpha)*x_ant + alpha*u;
% 
%     x_ant = saida_filtro;
%         
% 
%     saida_filtro = x_ant;
% 
%     
% end

== matlab function obs_com_filtro_2020/Dist_Observer5/Statistic Filter ==
  settings: updateMethod=DISCRETE
  data: u input; saida_filtro output; std_dev parameter; alpha output
%Autor: Lucas Moura Gomes
%Filtro estatístico.

function [saida_filtro, alpha]  = filtroPID( u, std_dev)
    persistent x_ant;
    persistent alpha_orig;
    
    if isempty(x_ant)
        x_ant = 0;
        Ts = 0.01; %sampling time
        tf = 2; %continuous time cte.
        alpha_orig = 1 - exp(-1/tf * Ts); %c2d filter
    end
    
    alpha = erf(abs(x_ant - u)/(sqrt(2)*2*std_dev));
    
    if alpha > 1
        alpha = 1;
    end
    
    %up = 1.1; %upper bound 10%
    %alpha = alpha * alpha_orig * up;
    
    saida_filtro = (1-alpha)*x_ant + alpha*u;
    
    x_ant = saida_filtro;
end

%Autor: Lucas Moura Gomes
%Filtro estatístico.
% 
% function [saida_filtro, alpha] = filtroPID( u, erro_tipico_medicao, Tf  )
% 	
%     persistent x_ant;
%     
%     if isempty(x_ant)
%         x_ant = 0;
%     end
%     
%     Tf = Tf/1.5;
%     a_Tf = 1 - exp(-1/Tf * 5);
%     
%     alpha = erf(abs(x_ant - u)/(sqrt(2)*2*erro_tipico_medicao));
%     
%     if alpha > 1 
%         alpha = 1;
%     end;
%     
%     saida_filtro = (1-alpha)*x_ant + alpha*u;
% 
%     x_ant = saida_filtro;
%         
% 
%     saida_filtro = x_ant;
% 
%     
% end

== matlab function obs_com_filtro_2020/Dist_Observer7/Statistic Filter ==
  settings: updateMethod=DISCRETE
  data: u input; saida_filtro output; std_dev parameter; alpha output
%Autor: Lucas Moura Gomes
%Filtro estatístico.

function [saida_filtro, alpha]  = filtroPID( u, std_dev)
    persistent x_ant;
    persistent alpha_orig;
    
    if isempty(x_ant)
        x_ant = 0;
        Ts = 0.01; %sampling time
        tf = 2; %continuous time cte.
        alpha_orig = 1 - exp(-1/tf * Ts); %c2d filter
    end
    
    alpha = erf(abs(x_ant - u)/(sqrt(2)*2*std_dev));
    
    if alpha > 1
        alpha = 1;
    end
    
    %up = 1.1; %upper bound 10%
    %alpha = alpha * alpha_orig * up;
    
    saida_filtro = (1-alpha)*x_ant + alpha*u;
    
    x_ant = saida_filtro;
end

%Autor: Lucas Moura Gomes
%Filtro estatístico.
% 
% function [saida_filtro, alpha] = filtroPID( u, erro_tipico_medicao, Tf  )
% 	
%     persistent x_ant;
%     
%     if isempty(x_ant)
%         x_ant = 0;
%     end
%     
%     Tf = Tf/1.5;
%     a_Tf = 1 - exp(-1/Tf * 5);
%     
%     alpha = erf(abs(x_ant - u)/(sqrt(2)*2*erro_tipico_medicao));
%     
%     if alpha > 1 
%         alpha = 1;
%     end;
%     
%     saida_filtro = (1-alpha)*x_ant + alpha*u;
% 
%     x_ant = saida_filtro;
%         
% 
%     saida_filtro = x_ant;
% 
%     
% end

== matlab function obs_com_filtro_2020/Dist_Observer8/Statistic Filter1 ==
  settings: updateMethod=DISCRETE
  data: u input; saida_filtro output; std_dev parameter; alpha output
%Autor: Lucas Moura Gomes
%Filtro estatístico.

function [saida_filtro, alpha]  = filtroPID( u, std_dev)
    persistent x_ant;
    persistent alpha_orig;
    
    if isempty(x_ant)
        x_ant = 0;
        Ts = 0.01; %sampling time
        tf = 2; %continuous time cte.
        alpha_orig = 1 - exp(-1/tf * Ts); %c2d filter
    end
    
    alpha = erf(abs(x_ant - u)/(sqrt(2)*2*std_dev));
    
    if alpha > 1
        alpha = 1;
    end
    
    %up = 1.1; %upper bound 10%
    %alpha = alpha * alpha_orig * up;
    
    saida_filtro = (1-alpha)*x_ant + alpha*u;
    
    x_ant = saida_filtro;
end

%Autor: Lucas Moura Gomes
%Filtro estatístico.
% 
% function [saida_filtro, alpha] = filtroPID( u, erro_tipico_medicao, Tf  )
% 	
%     persistent x_ant;
%     
%     if isempty(x_ant)
%         x_ant = 0;
%     end
%     
%     Tf = Tf/1.5;
%     a_Tf = 1 - exp(-1/Tf * 5);
%     
%     alpha = erf(abs(x_ant - u)/(sqrt(2)*2*erro_tipico_medicao));
%     
%     if alpha > 1 
%         alpha = 1;
%     end;
%     
%     saida_filtro = (1-alpha)*x_ant + alpha*u;
% 
%     x_ant = saida_filtro;
%         
% 
%     saida_filtro = x_ant;
% 
%     
% end

== matlab function obs_com_filtro_2020/Dist_Observer10/Statistic Filter ==
  settings: updateMethod=DISCRETE
  data: u input; saida_filtro output; std_dev parameter; alpha output
%Autor: Lucas Moura Gomes
%Filtro estatístico.

function [saida_filtro, alpha]  = filtroPID( u, std_dev)
    persistent x_ant;
    persistent alpha_orig;
    
    if isempty(x_ant)
        x_ant = 0;
        Ts = 0.01; %sampling time
        tf = 2; %continuous time cte.
        alpha_orig = 1 - exp(-1/tf * Ts); %c2d filter
    end
    
    alpha = erf(abs(x_ant - u)/(sqrt(2)*2*std_dev));
    
    if alpha > 1
        alpha = 1;
    end
    
    %up = 1.1; %upper bound 10%
    %alpha = alpha * alpha_orig * up;
    
    saida_filtro = (1-alpha)*x_ant + alpha*u;
    
    x_ant = saida_filtro;
end

%Autor: Lucas Moura Gomes
%Filtro estatístico.
% 
% function [saida_filtro, alpha] = filtroPID( u, erro_tipico_medicao, Tf  )
% 	
%     persistent x_ant;
%     
%     if isempty(x_ant)
%         x_ant = 0;
%     end
%     
%     Tf = Tf/1.5;
%     a_Tf = 1 - exp(-1/Tf * 5);
%     
%     alpha = erf(abs(x_ant - u)/(sqrt(2)*2*erro_tipico_medicao));
%     
%     if alpha > 1 
%         alpha = 1;
%     end;
%     
%     saida_filtro = (1-alpha)*x_ant + alpha*u;
% 
%     x_ant = saida_filtro;
%         
% 
%     saida_filtro = x_ant;
% 
%     
% end
